simulink model "q_rotpen_swingup_student"  (R2018b)
settings: Solver=ode1  StartTime=0.0  StopTime=inf  FixedStep=0.002  RelTol=1e-3  EnableMultiTasking=on
PostLoadFcn:
  | qc_set_target_type(getConfigSet(bdroot, 'QUARC Default Target Configuration'));
values from neighbouring files (symbols this model uses):
  epsilon = 12.0 * pi / 180    (= 0.209439510239)    [Linearization.m]
  Er = Mp*g*Lp    (= 0.4192975485)    [Linearization.m]
  eta_g = 0.90    (= 0.9)    [Linearization.m]
  eta_m = 0.69    [Linearization.m]
  g = 9.81    [Linearization.m]
  Jp = Mp*Lp^2/12    (= 0.00119873080146)    [Linearization.m]
  K = acker(A, B, poles)    [Control_FurutaPendulum.m]    (also in Linearization.m = Control_FurutaPendulum(A,B,zeta,wn,p3,p4))
  K_AMP = 1    [Linearization.m]
  K_ENC = 2 * pi / ( 4 * 1024 )    (= 0.00153398078789)    [Linearization.m]
  Kg = Kgi * Kge    (= 70)    [Linearization.m]
  km = 0.804 / 1000 * (60 / ( 2 * pi ))    (= 0.00767763445475)    [Linearization.m]
  kt = 1.088 * 0.2780139 * 0.0254    (= 0.00768296972928)    [Linearization.m]
  Lp = 0.33655    [Linearization.m]
  Lr = 0.2159    [Linearization.m]
  Mp = 0.127    [Linearization.m]
  Mr = 0.257    [Linearization.m]
  Rm = 2.6    [Linearization.m]
  wcf_1 = 2 * pi * 10.0    (= 62.8318530718)    [Linearization.m]
  wcf_2 = 2 * pi * 10.0    (= 62.8318530718)    [Linearization.m]
libraries: simulink_extras x3, simulink x3
settings Model: SimulationMode=external  ExtModeTrigDuration=10000  Creator=MLevis  LastModifiedBy=Joe Overcashier
settings SolverCC: PositivePriorityOrder=on
settings DataIOCC: LimitDataPoints=on  SaveFormat=Array  SignalLoggingSaveFormat=ModelDataLogs
settings OptimizationCC: ExpressionDepthLimit=2147483647  InitFltsAndDblsToZero=on  LifeSpan=inf
settings DebuggingCC: SaveWithParameterizedLinksMsg=none  UnderspecifiedInitializationDetection=Classic  MergeDetectMultiDrivingBlocksExec=none  SolverPrmCheckMsg=warning  MultiTaskDSMMsg=warning  MultiTaskCondExecSysMsg=none  FcnCallInpInsideContextMsg=warning  StateNameClashWarn=warning  SFUnexpectedBacktrackingDiag=warning  SFNoUnconditionalDefaultTransitionDiag=warning  SFExecutionAtInitializationDiag=none
settings HardwareCC: ProdBitPerPointer=32  ProdBitPerSizeT=32  ProdBitPerPtrDiffT=32  ProdLargestAtomicFloat=None  ProdIntDivRoundTo=Undefined  ProdEndianess=Unspecified  ProdWordSize=32  ProdHWDeviceType=32-bit Generic
settings ModelReferenceCC: PropagateSignalLabelsOutOfModel=off
settings SFSimCC: SimUseLocalCustomCode=off
settings RTWCC: SystemTargetFile=quarc_win64.tlc  TemplateMakefile=quarc_default_tmf  Description=QUARC Win64 Target  RTWUseLocalCustomCode=off
settings CodeAppCC: StateflowObjectComments=on
settings STFCustomTargetCC: TargetPreCompLibLocation=C:\PROGRA~3\QUARC\lib\2018b\win64\release  GeneratePreprocessorConditionals=Disable all  CPPClassGenCompliant=on  GRTInterface=on  SystemTargetFile=quarc_win64.tlc
settings GRTTargetCC: TargetPreCompLibLocation=C:\PROGRA~3\QUARC\lib\2018b\win64\release  TargetLangStandard=C89/C90 (ANSI)  ParMdlRefBuildCompliant=off  CompOptLevelCompliant=off  ConcurrentExecutionCompliant=off  GeneratePreprocessorConditionals=Disable all  CombineOutputUpdateFcns=off  MatFileLogging=off  GRTInterface=on  UseToolchainInfoCompliant=off  ExtMode=on  ExtModeMexFile=quarc_comm
settings ConfigComp: CovMetricSettings=dw  CovHtmlReporting=on  CovSaveCumulativeToWorkspaceVar=on  CovSaveSingleToWorkspaceVar=on  CovExternalEMLEnable=off

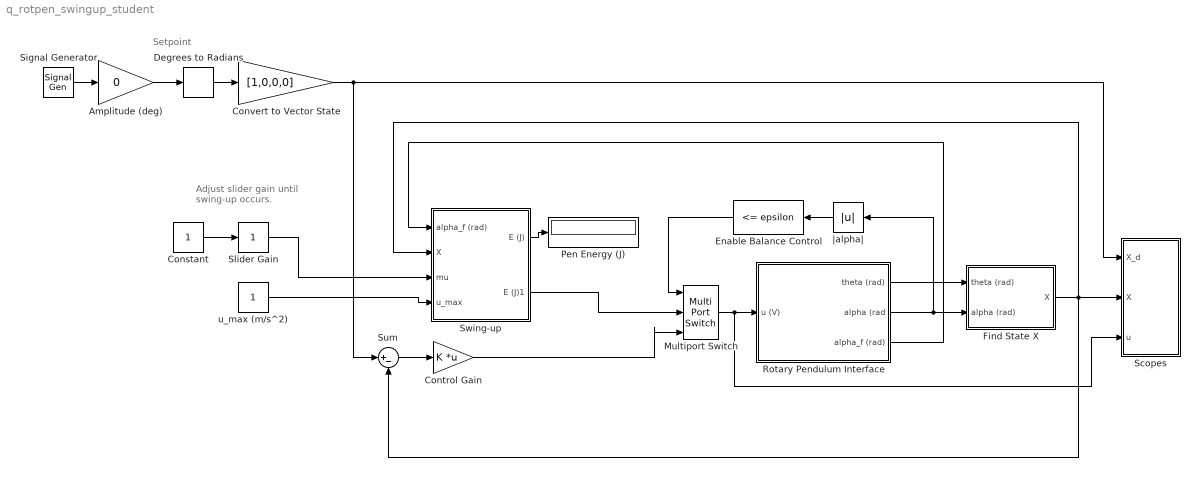
== system q_rotpen_swingup_student ==
  note: Setpoint
  note: Adjust slider gain
      | until swing-up occurs.
  Amplitude (deg) : Gain  Gain=0  SaturateOnIntegerOverflow=on  OutDataTypeStr=Inherit: Same as input  ParamDataTypeStr=Inherit: Same as input
  Constant : Constant
  Control Gain : Gain  Gain=K  Multiplication=Matrix(K*u)
  Convert to Vector State : Gain  Gain=[1,0,0,0]
  Degrees to Radians : simulink_extras/Transformations/Degrees to Radians
  Enable Balance Control : simulink/Logic and Bit Operations/Compare To Constant  relop=<=  const=epsilon  OutDataTypeStr=uint8  ZeroCross=off
  Find State X : Subsystem
  Multiport Switch : MultiPortSwitch  Inputs=2
  Pen Energy (J) : Display
      settings: Decimation=100
  Rotary Pendulum Interface : Subsystem
  Scopes : Subsystem
  Signal Generator : SignalGenerator  WaveForm=square  Frequency=0.1
  Slider Gain : simulink/Math Operations/Slider Gain  gain=1  low=0  high=10
  Sum : Sum  Inputs=|+-
  Swing-up : Subsystem
  u_max (m/s^2) : Constant
  |alpha| : Abs
  wires:
  Amplitude (deg)/1 -> Degrees to Radians/1
  Signal Generator/1 -> Amplitude (deg)/1
  Degrees to Radians/1 -> Convert to Vector State/1
  Convert to Vector State/1 -> Scopes/1(X_d), Sum/1
  Find State X/1(X) -> Scopes/2(X), Sum/2, Swing-up/2(X)
  Rotary Pendulum Interface/1(theta (rad)) -> Find State X/1(theta (rad))
  Rotary Pendulum Interface/2(alpha (rad) -> Find State X/2(alpha (rad)), |alpha|/1
  Sum/1 -> Control Gain/1
  |alpha|/1 -> Enable Balance Control/1
  Rotary Pendulum Interface/3(alpha_f (rad)) -> Swing-up/1(alpha_f (rad))
  Constant/1 -> Slider Gain/1
  Slider Gain/1 -> Swing-up/3(mu)
  Swing-up/1(E (J)) -> Pen Energy (J)/1
  u_max (m/s^2)/1 -> Swing-up/4(u_max)
  Multiport Switch/1 -> Rotary Pendulum Interface/1(u (V)), Scopes/3(u)
  Enable Balance Control/1 -> Multiport Switch/1
  Control Gain/1 -> Multiport Switch/3
  Swing-up/2(E (J)1) -> Multiport Switch/2

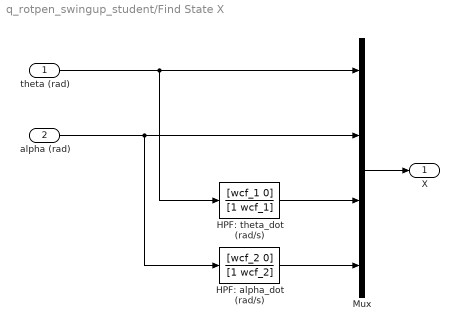
== system q_rotpen_swingup_student/Find State X ==
  theta (rad) : Inport
  alpha (rad) : Inport  Port=2
  HPF: alpha_dot (rad/s) : TransferFcn  Numerator=[wcf_2 0]  Denominator=[1 wcf_2]
  HPF: theta_dot (rad/s) : TransferFcn  Numerator=[wcf_1 0]  Denominator=[1 wcf_1]
  Mux : Mux
  X : Outport
  wires:
  alpha (rad)/1 -> Mux/2, HPF: alpha_dot (rad/s)/1
  Mux/1 -> X/1
  theta (rad)/1 -> Mux/1, HPF: theta_dot (rad/s)/1
  HPF: theta_dot (rad/s)/1 -> Mux/3
  HPF: alpha_dot (rad/s)/1 -> Mux/4

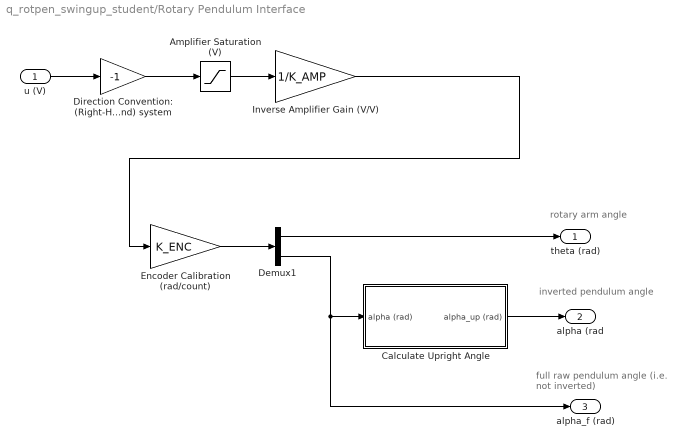
== system q_rotpen_swingup_student/Rotary Pendulum Interface ==
  note: full raw pendulum angle
      |  (i.e. not inverted)
  note: rotary arm angle
  note: inverted pendulum angle
  u (V) : Inport
  Amplifier Saturation (V) : Saturate  UpperLimit=5  LowerLimit=-5
  Calculate Upright Angle : Subsystem
  Demux1 : Demux  Outputs=2
  Direction Convention: (Right-Hand) system : Gain  Gain=-1  SaturateOnIntegerOverflow=on  OutDataTypeStr=Inherit: Same as input  ParamDataTypeStr=Inherit: Same as input
  Encoder Calibration (rad/count) : Gain  Gain=K_ENC  SaturateOnIntegerOverflow=on  OutDataTypeStr=Inherit: Same as input  ParamDataTypeStr=Inherit: Same as input
  Inverse Amplifier Gain (V/V) : Gain  Gain=1/K_AMP
  theta (rad) : Outport
  alpha (rad : Outport  Port=2
  alpha_f (rad) : Outport  Port=3
  wires:
  Calculate Upright Angle/1(alpha_up (rad)) -> alpha (rad/1
  Demux1/1 -> theta (rad)/1
  Direction Convention: (Right-Hand) system/1 -> Amplifier Saturation (V)/1
  u (V)/1 -> Direction Convention: (Right-Hand) system/1
  Amplifier Saturation (V)/1 -> Inverse Amplifier Gain (V/V)/1
  Inverse Amplifier Gain (V/V)/1 -> Encoder Calibration (rad/count)/1
  Demux1/2 -> alpha_f (rad)/1, Calculate Upright Angle/1(alpha (rad))
  Encoder Calibration (rad/count)/1 -> Demux1/1

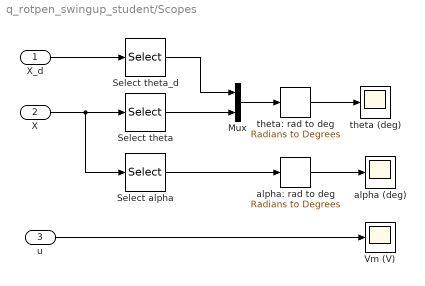
== system q_rotpen_swingup_student/Scopes ==
  X_d : Inport
  X : Inport  Port=2
  u : Inport  Port=3
  Mux : Mux  Inputs=2
  Select alpha : Selector  InputPortWidth=4  IndexOptions=Index vector (dialog)  Indices=2  OutputSizes=[(-2)]
  Select theta : Selector  InputPortWidth=4  IndexOptions=Index vector (dialog)  Indices=1  OutputSizes=[(-2)]
  Select theta_d : Selector  InputPortWidth=4  IndexOptions=Index vector (dialog)  Indices=1  OutputSizes=[(-2)]
  Vm (V) : Scope
  alpha (deg) : Scope
  alpha: rad to deg : simulink_extras/Transformations/Radians to Degrees
  theta (deg) : Scope
  theta: rad to deg : simulink_extras/Transformations/Radians to Degrees
  wires:
  u/1 -> Vm (V)/1
  X_d/1 -> Select theta_d/1
  Mux/1 -> theta: rad to deg/1
  Select alpha/1 -> alpha: rad to deg/1
  alpha: rad to deg/1 -> alpha (deg)/1
  X/1 -> Select alpha/1, Select theta/1
  Select theta_d/1 -> Mux/1
  theta: rad to deg/1 -> theta (deg)/1
  Select theta/1 -> Mux/2

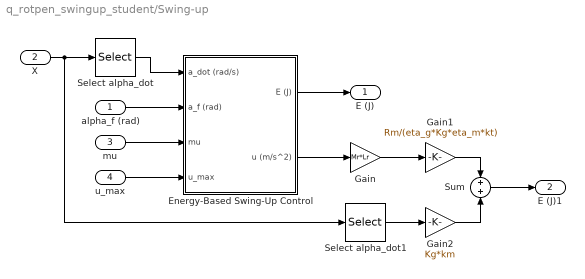
== system q_rotpen_swingup_student/Swing-up ==
  alpha_f (rad) : Inport
  X : Inport  Port=2
  mu : Inport  Port=3
  u_max : Inport  Port=4
  Energy-Based Swing-Up Control : Subsystem
  Gain : Gain  Gain=Mr*Lr
  Gain1 : Gain  Gain=Rm/(eta_g*Kg*eta_m*kt)
  Gain2 : Gain  Gain=Kg*km
  Select alpha_dot : Selector  InputPortWidth=4  IndexOptions=Index vector (dialog)  Indices=[4]  OutputSizes=1
  Select alpha_dot1 : Selector  InputPortWidth=4  IndexOptions=Index vector (dialog)  Indices=[3]  OutputSizes=1
  Sum : Sum
  E (J) : Outport
  E (J)1 : Outport  Port=2
  wires:
  Energy-Based Swing-Up Control/1(E (J)) -> E (J)/1
  alpha_f (rad)/1 -> Energy-Based Swing-Up Control/2(a_f (rad))
  mu/1 -> Energy-Based Swing-Up Control/3(mu)
  Select alpha_dot/1 -> Energy-Based Swing-Up Control/1(a_dot (rad/s))
  X/1 -> Select alpha_dot1/1, Select alpha_dot/1
  u_max/1 -> Energy-Based Swing-Up Control/4(u_max)
  Energy-Based Swing-Up Control/2(u (m/s^2)) -> Gain/1
  Gain/1 -> Gain1/1
  Select alpha_dot1/1 -> Gain2/1
  Gain1/1 -> Sum/1
  Gain2/1 -> Sum/2
  Sum/1 -> E (J)1/1

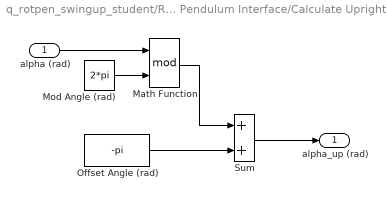
== system q_rotpen_swingup_student/Rotary Pendulum Interface/Calculate Upright Angle ==
  alpha (rad) : Inport
  Math Function : Math  Operator=mod  SaturateOnIntegerOverflow=on
  Mod Angle (rad) : Constant  Value=2*pi
  Offset Angle (rad) : Constant  Value=-pi
  Sum : Sum  SaturateOnIntegerOverflow=on  InputSameDT=on  OutDataTypeStr=Inherit: Same as first input
  alpha_up (rad) : Outport
  wires:
  Math Function/1 -> Sum/1
  alpha (rad)/1 -> Math Function/1
  Offset Angle (rad)/1 -> Sum/2
  Mod Angle (rad)/1 -> Math Function/2
  Sum/1 -> alpha_up (rad)/1

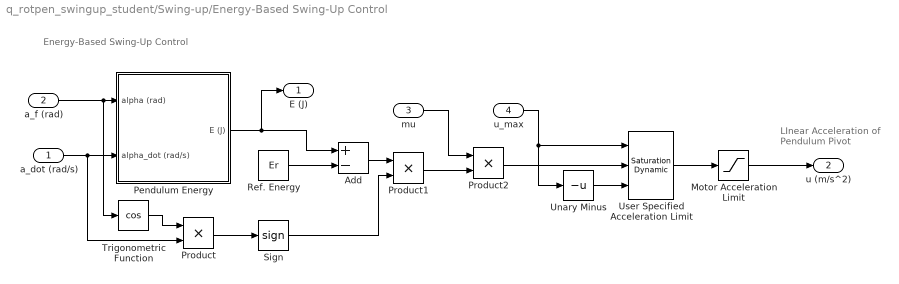
== system q_rotpen_swingup_student/Swing-up/Energy-Based Swing-Up Control ==
  note: Energy-Based Swing-Up Control
  note: LInear Acceleration of
      | Pendulum Pivot
  a_dot (rad/s) : Inport
  a_f (rad) : Inport  Port=2
  mu : Inport  Port=3
  u_max : Inport  Port=4
  Add : Sum  Inputs=+-
  Motor Acceleration Limit : Saturate  UpperLimit=10  LowerLimit=-10
  Pendulum Energy : Subsystem
  Product : Product
  Product1 : Product
  Product2 : Product
  Ref. Energy : Constant  Value=Er
  Sign : Signum
  Trigonometric Function : Trigonometry  Operator=cos
  Unary Minus : UnaryMinus
  User Specified Acceleration Limit : simulink/Discontinuities/Saturation Dynamic  OutMin=[]  OutMax=[]  OutDataTypeStr=Inherit: Same as second input  OutDataType=fixdt(1, 16)  OutScaling=2^-10  DoSatur=off
  E (J) : Outport
  u (m/s^2) : Outport  Port=2
  wires:
  a_f (rad)/1 -> Trigonometric Function/1, Pendulum Energy/1(alpha (rad))
  Pendulum Energy/1(E (J)) -> Add/1, E (J)/1
  Product2/1 -> User Specified Acceleration Limit/2
  u_max/1 -> User Specified Acceleration Limit/1, Unary Minus/1
  Unary Minus/1 -> User Specified Acceleration Limit/3
  User Specified Acceleration Limit/1 -> Motor Acceleration Limit/1
  Motor Acceleration Limit/1 -> u (m/s^2)/1
  Trigonometric Function/1 -> Product/1
  a_dot (rad/s)/1 -> Product/2, Pendulum Energy/2(alpha_dot (rad/s))
  Product/1 -> Sign/1
  Ref. Energy/1 -> Add/2
  Add/1 -> Product1/1
  Sign/1 -> Product1/2
  Product1/1 -> Product2/2
  mu/1 -> Product2/1

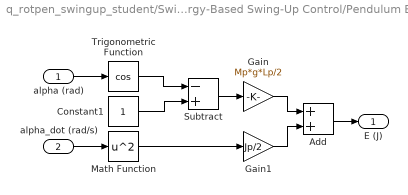
== system q_rotpen_swingup_student/Swing-up/Energy-Based Swing-Up Control/Pendulum Energy ==
  alpha (rad) : Inport
  alpha_dot (rad/s) : Inport  Port=2
  Add : Sum
  Constant1 : Constant
  Gain : Gain  Gain=Mp*g*Lp/2
  Gain1 : Gain  Gain=Jp/2
  Math Function : Math  Operator=square  SaturateOnIntegerOverflow=on
  Subtract : Sum  Inputs=-+
  Trigonometric Function : Trigonometry  Operator=cos
  E (J) : Outport
  wires:
  Add/1 -> E (J)/1
  alpha (rad)/1 -> Trigonometric Function/1
  Constant1/1 -> Subtract/2
  Subtract/1 -> Gain/1
  Gain/1 -> Add/1
  alpha_dot (rad/s)/1 -> Math Function/1
  Gain1/1 -> Add/2
  Math Function/1 -> Gain1/1
  Trigonometric Function/1 -> Subtract/1
